simulink model "main_signal_system"  (R2025b)
settings: Solver=VariableStepAuto  StartTime=0.0  StopTime=10.0  RelTol=1e-3
libraries: commhdlcrc x3, hdlsllib x3, simulink x2
settings Model: Creator=strog  LastModifiedBy=strog
settings OptimizationCC: BlockReduction=off  ConditionallyExecuteInputs=off

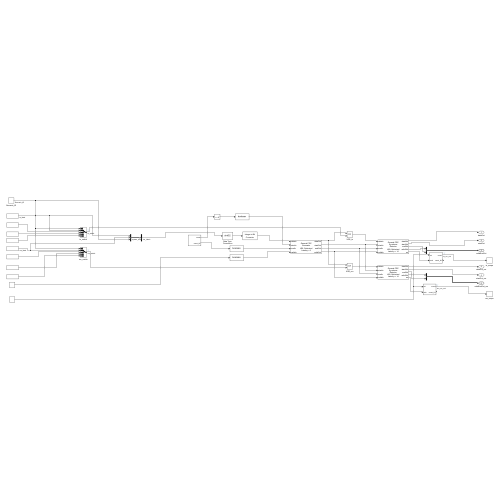
[thumbnail: Simulink's stored preview of the top-level diagram]
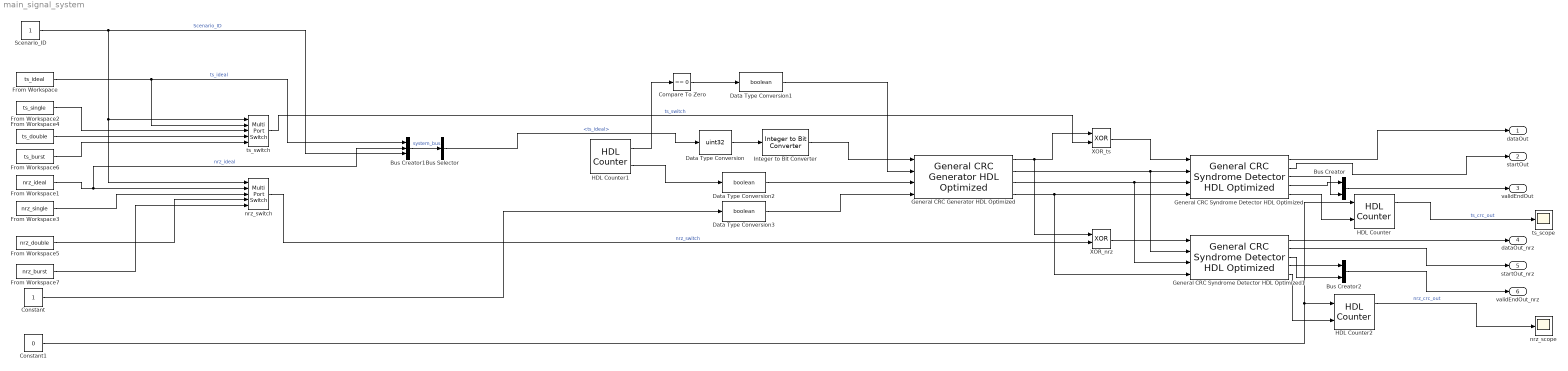
== system main_signal_system ==
  Bus Creator : BusCreator  Inputs=2
  Bus Creator1 : BusCreator  Inputs=3
  Bus Creator2 : BusCreator  Inputs=2
  Bus Selector : BusSelector  OutputSignals=ts_ideal
  Compare To Zero : simulink/Logic and Bit Operations/Compare To Zero  relop===  OutDataTypeStr=boolean
  Constant : Constant
  Constant1 : Constant  Value=0  OutDataTypeStr=boolean
  Data Type Conversion : DataTypeConversion  OutDataTypeStr=uint32  SaturateOnIntegerOverflow=off  RndMeth=Floor
  Data Type Conversion1 : DataTypeConversion  OutDataTypeStr=boolean  SaturateOnIntegerOverflow=off  RndMeth=Floor
  Data Type Conversion2 : DataTypeConversion  OutDataTypeStr=boolean  SaturateOnIntegerOverflow=off  RndMeth=Floor
  Data Type Conversion3 : DataTypeConversion  OutDataTypeStr=boolean  SaturateOnIntegerOverflow=off  RndMeth=Floor
  From Workspace : FromWorkspace  VariableName=ts_ideal
  From Workspace1 : FromWorkspace  VariableName=nrz_ideal
  From Workspace2 : FromWorkspace  VariableName=ts_single
  From Workspace3 : FromWorkspace  VariableName=nrz_single
  From Workspace4 : FromWorkspace  VariableName=ts_double
  From Workspace5 : FromWorkspace  VariableName=nrz_double
  From Workspace6 : FromWorkspace  VariableName=ts_burst
  From Workspace7 : FromWorkspace  VariableName=nrz_burst
  General CRC Generator HDL Optimized : commhdlcrc/General CRC Generator HDL Optimized  Polynomial=polyCoeffs  InitialState=1  DirectMethod=on  ReflectInput=on  ReflectCRCChecksum=on  FinalXORValue=ones(1, 32)  SimulateUsing=Code generation
  General CRC Syndrome Detector HDL Optimized : commhdlcrc/General CRC Syndrome Detector HDL Optimized  Polynomial=polyCoeffs  InitialState=1  DirectMethod=on  ReflectInput=on  ReflectCRCChecksum=on  FinalXORValue=ones(1, 32)  SimulateUsing=Code generation
  General CRC Syndrome Detector HDL Optimized1 : commhdlcrc/General CRC Syndrome Detector HDL Optimized  Polynomial=polyCoeffs  InitialState=1  DirectMethod=on  ReflectInput=on  ReflectCRCChecksum=on  FinalXORValue=ones(1, 32)  SimulateUsing=Code generation
  HDL Counter : hdlsllib/Sources/HDL Counter  CountType=Count limited  CountInit=0  CountStep=1  CountMax=25  CountFromType=Initial value  CountFrom=0  CountResetPort=on  CountLoadPort=off  CountEnbPort=on  CountDirPort=off  CountHitOutputPort=on  CountDataType=Unsigned  CountWordLen=8  CountFracLen=0  CountSampTime=uint8(1)
  HDL Counter1 : hdlsllib/Sources/HDL Counter  CountType=Count limited  CountInit=0  CountStep=1  CountMax=4  CountFromType=Initial value  CountFrom=0  CountResetPort=off  CountLoadPort=off  CountEnbPort=off  CountDirPort=off  CountHitOutputPort=on  CountDataType=Unsigned  CountWordLen=8  CountFracLen=0  CountSampTime=1
  HDL Counter2 : hdlsllib/Sources/HDL Counter  CountType=Count limited  CountInit=0  CountStep=1  CountMax=25  CountFromType=Initial value  CountFrom=0  CountResetPort=on  CountLoadPort=off  CountEnbPort=on  CountDirPort=off  CountHitOutputPort=on  CountDataType=Unsigned  CountWordLen=8  CountFracLen=0  CountSampTime=uint8(1)
  Integer to Bit Converter : simulink/Logic and Bit Operations/Integer to Bit Converter  nbits=8  signedInputValues=Unsigned  bitOrder=MSB first  outDtype=boolean
      settings: LibrarySourceBlock=|
      | commutil2/Integer to Bit
      | Converter
  Scenario_ID : Constant
  XOR_nrz : Logic  Operator=XOR  AllPortsSameDT=off  OutDataTypeStr=boolean
  XOR_ts : Logic  Operator=XOR  AllPortsSameDT=off  OutDataTypeStr=boolean
  nrz_scope : Scope
      settings: ActiveDisplayYMinimum=-42.821406355413558  ActiveDisplayYMaximum=21.216899971653731  DataLoggingSaveFormat=Array
  nrz_switch : MultiPortSwitch  Inputs=4  SaturateOnIntegerOverflow=off  InputSameDT=off
  ts_scope : Scope
      settings: ActiveDisplayYMinimum=-42.821406355413558  ActiveDisplayYMaximum=21.216899971653731  DataLoggingSaveFormat=Array
  ts_switch : MultiPortSwitch  Inputs=4  SaturateOnIntegerOverflow=off  InputSameDT=off
  dataOut : Outport
  startOut : Outport  Port=2
  validEndOut : Outport  Port=3  OutDataTypeStr=Bus: CRCStatusBus
  dataOut_nrz : Outport  Port=4
  startOut_nrz : Outport  Port=5
  validEndOut_nrz : Outport  Port=6  OutDataTypeStr=Bus: CRCStatusBus
  wires:
  Data Type Conversion3/1 -> General CRC Generator HDL Optimized/4
  HDL Counter1/2 -> Data Type Conversion2/1
  General CRC Syndrome Detector HDL Optimized/1 -> dataOut/1
  HDL Counter1/1 -> Compare To Zero/1
  Constant1/1 -> HDL Counter2/1, HDL Counter/1
  General CRC Syndrome Detector HDL Optimized/2 -> startOut/1
  Compare To Zero/1 -> Data Type Conversion1/1
  Data Type Conversion2/1 -> General CRC Generator HDL Optimized/3
  General CRC Syndrome Detector HDL Optimized/3 -> Bus Creator/2
  General CRC Generator HDL Optimized/1 -> XOR_nrz/1, XOR_ts/1
  General CRC Syndrome Detector HDL Optimized/4 -> Bus Creator/1
  Data Type Conversion1/1 -> General CRC Generator HDL Optimized/2
  HDL Counter/1 -> ts_scope/1  "ts_crc_out"
  Bus Creator/1 -> validEndOut/1
  General CRC Generator HDL Optimized/2 -> General CRC Syndrome Detector HDL Optimized1/2, General CRC Syndrome Detector HDL Optimized/2
  General CRC Generator HDL Optimized/3 -> General CRC Syndrome Detector HDL Optimized1/3, General CRC Syndrome Detector HDL Optimized/3
  Integer to Bit Converter/1 -> General CRC Generator HDL Optimized/1
  XOR_ts/1 -> General CRC Syndrome Detector HDL Optimized/1
  From Workspace/1 -> Bus Creator1/1, ts_switch/2  "ts_ideal"
  From Workspace2/1 -> ts_switch/3
  From Workspace4/1 -> ts_switch/4
  From Workspace6/1 -> ts_switch/5
  From Workspace1/1 -> Bus Creator1/2, nrz_switch/2  "nrz_ideal"
  From Workspace3/1 -> nrz_switch/3
  From Workspace5/1 -> nrz_switch/4
  From Workspace7/1 -> nrz_switch/5
  Scenario_ID/1 -> ts_switch/1, nrz_switch/1, Bus Creator1/3  "Scenario_ID"
  Bus Creator1/1 -> Bus Selector/1  "system_bus"
  Data Type Conversion/1 -> Integer to Bit Converter/1
  General CRC Syndrome Detector HDL Optimized/5 -> HDL Counter/2
  ts_switch/1 -> XOR_ts/2  "ts_switch"
  Bus Selector/1 -> Data Type Conversion/1  "<ts_ideal>"
  nrz_switch/1 -> XOR_nrz/2  "nrz_switch"
  XOR_nrz/1 -> General CRC Syndrome Detector HDL Optimized1/1
  General CRC Syndrome Detector HDL Optimized1/1 -> dataOut_nrz/1
  HDL Counter2/1 -> nrz_scope/1  "nrz_crc_out"
  Bus Creator2/1 -> validEndOut_nrz/1
  General CRC Syndrome Detector HDL Optimized1/2 -> startOut_nrz/1
  General CRC Syndrome Detector HDL Optimized1/3 -> Bus Creator2/2
  General CRC Syndrome Detector HDL Optimized1/4 -> Bus Creator2/1
  General CRC Syndrome Detector HDL Optimized1/5 -> HDL Counter2/2
  Constant/1 -> Data Type Conversion3/1
  General CRC Generator HDL Optimized/4 -> General CRC Syndrome Detector HDL Optimized1/4, General CRC Syndrome Detector HDL Optimized/4
